simulink model "model"  (R2024b)
settings: Solver=ode4  StartTime=0.0  StopTime=1  FixedStep=0.0002  MaxStep=1e-4  RelTol=1e-3  EnableMultiTasking=on
undefined symbols (not defined in the file): rr, rs
libraries: spsRMSLib x1, simulink x1
settings Model: PacingRate=0.200000  Creator=jw  LastModifiedBy=tnt4
settings SolverCC: AlgebraicLoopSolver=TrustRegion
settings DataIOCC: LimitDataPoints=on  SaveFormat=Array  SignalLoggingSaveFormat=ModelDataLogs  ReturnWorkspaceOutputs=off
settings OptimizationCC: InitFltsAndDblsToZero=on  LifeSpan=inf
settings DebuggingCC: SaveWithParameterizedLinksMsg=none  UnderspecifiedInitializationDetection=Classic  MergeDetectMultiDrivingBlocksExec=none  SignalResolutionControl=TryResolveAllWithWarning  SolverPrmCheckMsg=warning  MultiTaskDSMMsg=warning  MultiTaskCondExecSysMsg=none  FcnCallInpInsideContextMsg=warning  UnconnectedInputMsg=warning  UnconnectedOutputMsg=warning  UnconnectedLineMsg=warning  SFUnexpectedBacktrackingDiag=warning  SFNoUnconditionalDefaultTransitionDiag=warning  SFExecutionAtInitializationDiag=none  ArithmeticOperatorsInVariantConditions=warning
settings HardwareCC: ProdBitPerPointer=32  ProdBitPerSizeT=32  ProdBitPerPtrDiffT=32  ProdLargestAtomicFloat=None  ProdIntDivRoundTo=Undefined  ProdEndianess=Unspecified  ProdWordSize=32  ProdHWDeviceType=32-bit Generic
settings ModelReferenceCC: EnableRefExpFcnMdlSchedulingChecks=on  PropagateSignalLabelsOutOfModel=off
settings SFSimCC: SimUseLocalCustomCode=off  CustomCodeUndefinedFunction=UseInterfaceOnly
settings RTWCC: RTWUseLocalCustomCode=off  GPUComputeCapability=3.5
settings CodeAppCC: StateflowObjectComments=on
settings GRTTargetCC: TargetFcnLib=ansi_tfl_tmw.mat  TargetLangStandard=C89/C90 (ANSI)  CombineOutputUpdateFcns=off  GRTInterface=on
settings ConfigComp: CovMetricSettings=dw  CovSaveCumulativeToWorkspaceVar=on  CovSaveSingleToWorkspaceVar=on  CovExternalEMLEnable=off

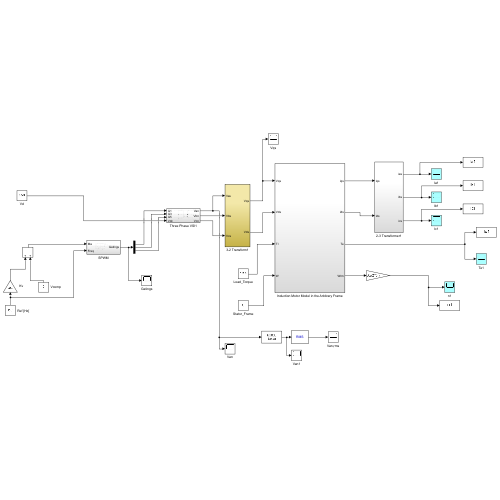
[thumbnail: Simulink's stored preview of the top-level diagram]
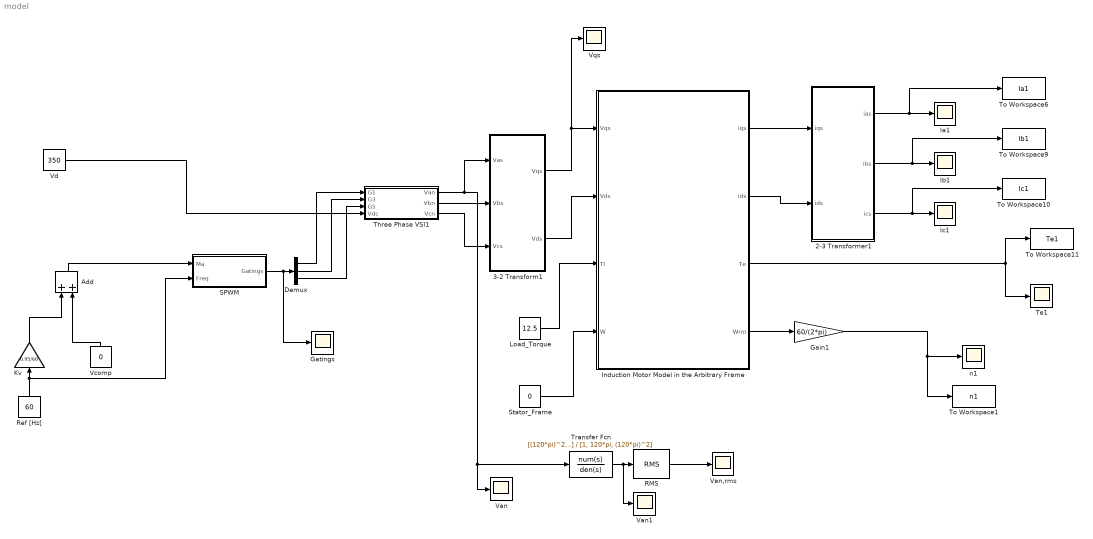
== system model ==
  2-3 Transformer1 : Subsystem
  3-2 Transform1 : Subsystem
  Add : Sum
  Demux : Demux  Outputs=3
  Gain1 : Gain  Gain=60/(2*pi)
  Gatings : Scope
  Ia1 : Scope
  Ib1 : Scope
  Ic1 : Scope
  Induction Motor Model in the Arbitrary Frame : Subsystem
  Kv : Gain  Gain=0.95/60
  Load_Torque : Constant  Value=12.5
  RMS : spsRMSLib/RMS  TrueRMS=on  Freq=60  RMSInit=0  Ts=0
  Ref [Hz[ : Constant  Value=60
  SPWM : Subsystem
  Stator_Frame : Constant  Value=0
  Te1 : Scope
  Three Phase VSI1 : Subsystem
  To Workspace1 : ToWorkspace  VariableName=n1  SampleTime=-1
  To Workspace10 : ToWorkspace  VariableName=Ic1  SampleTime=-1
  To Workspace11 : ToWorkspace  VariableName=Te1  SampleTime=-1
  To Workspace6 : ToWorkspace  VariableName=Ia1  SampleTime=-1
  To Workspace9 : ToWorkspace  VariableName=Ib1  SampleTime=-1
  Transfer Fcn : TransferFcn  Numerator=[(120*pi)^2]  Denominator=[1, 120*pi, (120*pi)^2]
  Van : Scope
  Van,rms : Scope
  Van1 : Scope
  Vcomp : Constant  Value=0
  Vd : Constant  Value=350
  Vqs : Scope
  n1 : Scope
  wires:
  Ref [Hz[/1 -> SPWM/2(Freq), Kv/1
  Kv/1 -> Add/1
  Vcomp/1 -> Add/2
  Add/1 -> SPWM/1(Ma)
  Vd/1 -> Three Phase VSI1/4(Vdc)
  SPWM/1(Gatings) -> Gatings/1, Demux/1
  Demux/1 -> Three Phase VSI1/1(G1)
  Demux/2 -> Three Phase VSI1/2(G3)
  Demux/3 -> Three Phase VSI1/3(G5)
  Three Phase VSI1/1(Van) -> Transfer Fcn/1, Van/1, 3-2 Transform1/1(Vas)
  Three Phase VSI1/2(Vbn) -> 3-2 Transform1/2(Vbs)
  Three Phase VSI1/3(Vcn) -> 3-2 Transform1/3(Vcs)
  3-2 Transform1/1(Vqs) -> Vqs/1, Induction Motor Model in the Arbitrary Frame/1(Vqs)
  3-2 Transform1/2(Vds) -> Induction Motor Model in the Arbitrary Frame/2(Vds)
  Stator_Frame/1 -> Induction Motor Model in the Arbitrary Frame/4(W)
  Load_Torque/1 -> Induction Motor Model in the Arbitrary Frame/3(Tl)
  Induction Motor Model in the Arbitrary Frame/1(iqs) -> 2-3 Transformer1/1(iqs)
  Induction Motor Model in the Arbitrary Frame/2(ids) -> 2-3 Transformer1/2(ids)
  Gain1/1 -> n1/1, To Workspace1/1
  Induction Motor Model in the Arbitrary Frame/4(Wrm) -> Gain1/1
  2-3 Transformer1/2(ibs) -> Ib1/1, To Workspace9/1
  2-3 Transformer1/3(ics) -> Ic1/1, To Workspace10/1
  2-3 Transformer1/1(ias) -> Ia1/1, To Workspace6/1
  Induction Motor Model in the Arbitrary Frame/3(Te) -> Te1/1, To Workspace11/1
  Transfer Fcn/1 -> Van1/1, RMS/1
  RMS/1 -> Van,rms/1

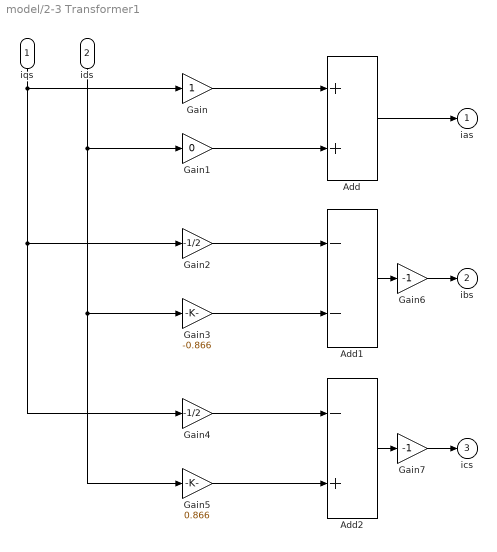
== system model/2-3 Transformer1 ==
  iqs : Inport
  ids : Inport  Port=2
  Add : Sum
  Add1 : Sum  Inputs=--
  Add2 : Sum  Inputs=-+
  Gain : Gain
  Gain1 : Gain  Gain=0
  Gain2 : Gain  Gain=-1/2
  Gain3 : Gain  Gain=-0.866
  Gain4 : Gain  Gain=-1/2
  Gain5 : Gain  Gain=0.866
  Gain6 : Gain  Gain=-1
  Gain7 : Gain  Gain=-1
  ias : Outport  InitialOutput=0  VectorParamsAs1DForOutWhenUnconnected=off
  ibs : Outport  Port=2  InitialOutput=0  VectorParamsAs1DForOutWhenUnconnected=off
  ics : Outport  Port=3  InitialOutput=0  VectorParamsAs1DForOutWhenUnconnected=off
  wires:
  Gain/1 -> Add/1
  Gain1/1 -> Add/2
  Gain2/1 -> Add1/1
  Gain3/1 -> Add1/2
  Gain4/1 -> Add2/1
  Gain5/1 -> Add2/2
  Add2/1 -> Gain7/1
  Add1/1 -> Gain6/1
  Add/1 -> ias/1
  iqs/1 -> Gain/1, Gain2/1, Gain4/1
  ids/1 -> Gain1/1, Gain3/1, Gain5/1
  Gain6/1 -> ibs/1
  Gain7/1 -> ics/1

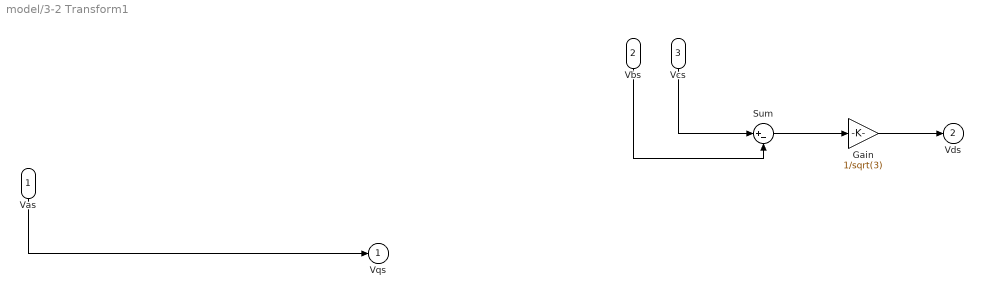
== system model/3-2 Transform1 ==
  Vas : Inport
  Vbs : Inport  Port=2
  Vcs : Inport  Port=3
  Gain : Gain  Gain=1/sqrt(3)
  Sum : Sum  Inputs=|+-
  Vqs : Outport  InitialOutput=0  VectorParamsAs1DForOutWhenUnconnected=off
  Vds : Outport  Port=2  InitialOutput=0  VectorParamsAs1DForOutWhenUnconnected=off
  wires:
  Vas/1 -> Vqs/1
  Vbs/1 -> Sum/2
  Vcs/1 -> Sum/1
  Sum/1 -> Gain/1
  Gain/1 -> Vds/1

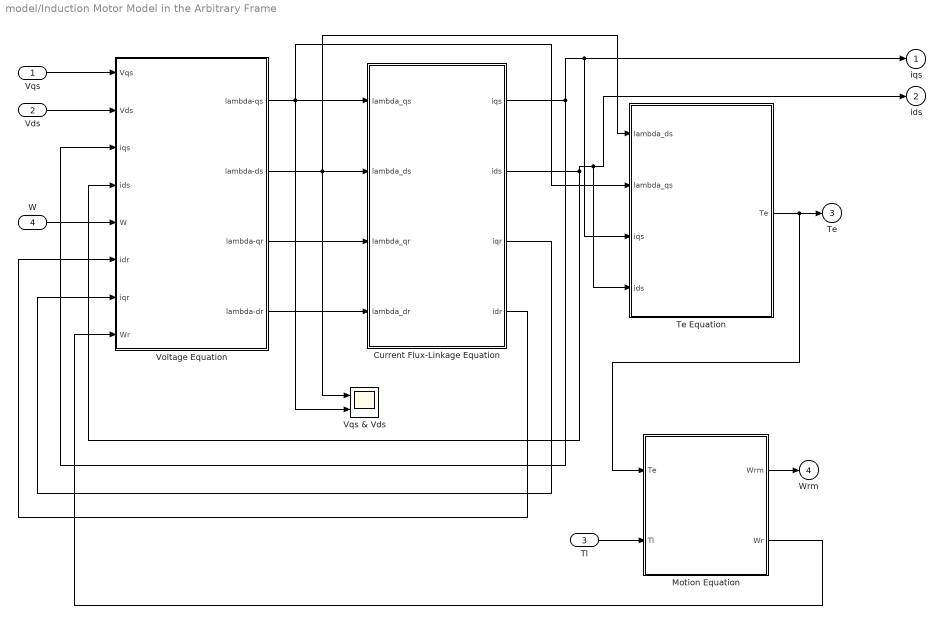
== system model/Induction Motor Model in the Arbitrary Frame ==
  Vqs : Inport
  Vds : Inport  Port=2
  Tl : Inport  Port=3
  W : Inport  Port=4
  Current Flux-Linkage Equation : Subsystem
  Motion Equation : Subsystem
  Te Equation : Subsystem
  Voltage Equation : Subsystem
  Vqs & Vds : Scope  NumInputPorts=2
  iqs : Outport  InitialOutput=0  VectorParamsAs1DForOutWhenUnconnected=off
  ids : Outport  Port=2  InitialOutput=0  VectorParamsAs1DForOutWhenUnconnected=off
  Te : Outport  Port=3  InitialOutput=0  VectorParamsAs1DForOutWhenUnconnected=off
  Wrm : Outport  Port=4  InitialOutput=0  VectorParamsAs1DForOutWhenUnconnected=off
  wires:
  Vqs/1 -> Voltage Equation/1(Vqs)
  Vds/1 -> Voltage Equation/2(Vds)
  Tl/1 -> Motion Equation/2(Tl)
  W/1 -> Voltage Equation/5(W)
  Te Equation/1(Te) -> Te/1, Motion Equation/1(Te)
  Current Flux-Linkage Equation/1(iqs) -> Voltage Equation/3(iqs), iqs/1, Te Equation/3(iqs)
  Current Flux-Linkage Equation/2(ids) -> Voltage Equation/4(ids), ids/1, Te Equation/4(ids)
  Current Flux-Linkage Equation/3(iqr) -> Voltage Equation/7(iqr)
  Voltage Equation/1(lambda-qs) -> Vqs & Vds/2, Current Flux-Linkage Equation/1(lambda_qs), Te Equation/2(lambda_qs)
  Voltage Equation/2(lambda-ds) -> Te Equation/1(lambda_ds), Vqs & Vds/1, Current Flux-Linkage Equation/2(lambda_ds)
  Voltage Equation/3(lambda-qr) -> Current Flux-Linkage Equation/3(lambda_qr)
  Voltage Equation/4(lambda-dr) -> Current Flux-Linkage Equation/4(lambda_dr)
  Current Flux-Linkage Equation/4(idr) -> Voltage Equation/6(idr)
  Motion Equation/2(Wr) -> Voltage Equation/8(Wr)
  Motion Equation/1(Wrm) -> Wrm/1

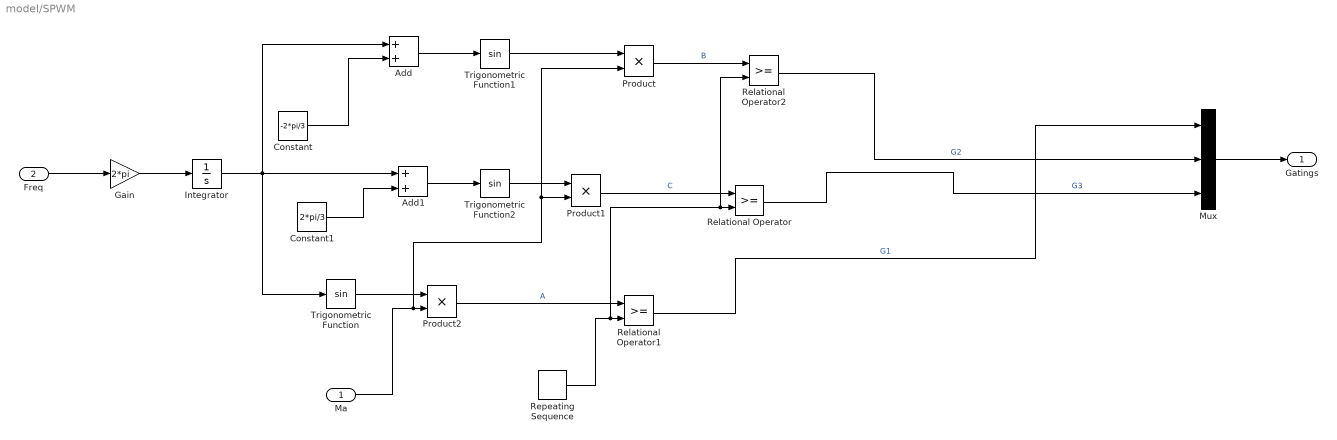
== system model/SPWM ==
  Ma : Inport
  Freq : Inport  Port=2
  Add : Sum
  Add1 : Sum
  Constant : Constant  Value=-2*pi/3
  Constant1 : Constant  Value=2*pi/3
  Gain : Gain  Gain=2*pi
  Integrator : Integrator
  Mux : Mux  Inputs=3
  Product : Product
  Product1 : Product
  Product2 : Product
  Relational Operator : RelationalOperator  OutDataTypeStr=boolean  RndMeth=Simplest  InputSameDT=off
  Relational Operator1 : RelationalOperator  OutDataTypeStr=boolean  RndMeth=Simplest  InputSameDT=off
  Relational Operator2 : RelationalOperator  OutDataTypeStr=boolean  RndMeth=Simplest  InputSameDT=off
  Repeating Sequence : simulink/Sources/Repeating Sequence  rep_seq_t=[0, 0.5/2000, 1/2000]  rep_seq_y=[-1, 1, -1]
  Trigonometric Function : Trigonometry
  Trigonometric Function1 : Trigonometry
  Trigonometric Function2 : Trigonometry
  Gatings : Outport
  wires:
  Integrator/1 -> Add1/1, Add/1, Trigonometric Function/1
  Ma/1 -> Product1/2, Product/2, Product2/2
  Gain/1 -> Integrator/1
  Add/1 -> Trigonometric Function1/1
  Trigonometric Function1/1 -> Product/1
  Trigonometric Function/1 -> Product2/1
  Add1/1 -> Trigonometric Function2/1
  Trigonometric Function2/1 -> Product1/1
  Constant/1 -> Add/2
  Constant1/1 -> Add1/2
  Freq/1 -> Gain/1
  Product/1 -> Relational Operator2/1  "B"
  Product1/1 -> Relational Operator/1  "C"
  Product2/1 -> Relational Operator1/1  "A"
  Repeating Sequence/1 -> Relational Operator2/2, Relational Operator/2, Relational Operator1/2
  Relational Operator1/1 -> Mux/1  "G1"
  Relational Operator2/1 -> Mux/2  "G2"
  Relational Operator/1 -> Mux/3  "G3"
  Mux/1 -> Gatings/1

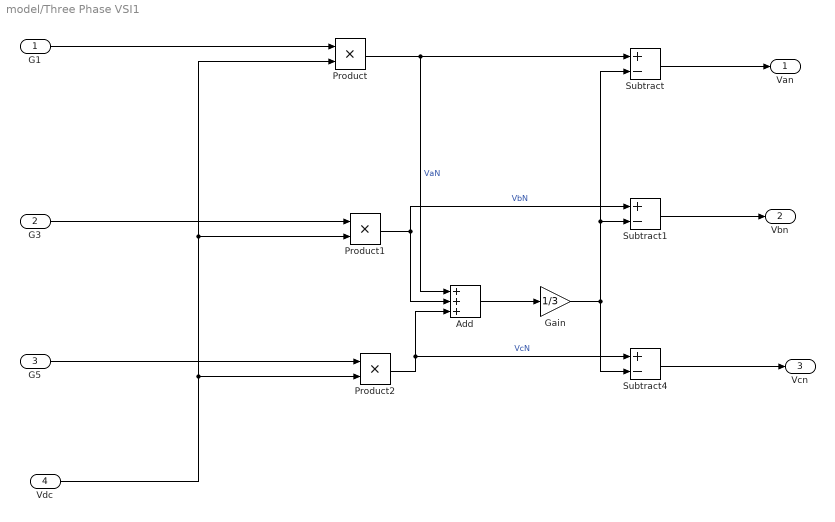
== system model/Three Phase VSI1 ==
  G1 : Inport
  G3 : Inport  Port=2
  G5 : Inport  Port=3
  Vdc : Inport  Port=4
  Add : Sum  Inputs=+++
  Gain : Gain  Gain=1/3
  Product : Product
  Product1 : Product
  Product2 : Product
  Subtract : Sum  Inputs=+-
  Subtract1 : Sum  Inputs=+-
  Subtract4 : Sum  Inputs=+-
  Van : Outport
  Vbn : Outport  Port=2
  Vcn : Outport  Port=3
  wires:
  G1/1 -> Product/1
  G3/1 -> Product1/1
  G5/1 -> Product2/1
  Vdc/1 -> Product2/2, Product1/2, Product/2
  Product/1 -> Subtract/1, Add/1  "VaN"
  Product1/1 -> Add/2, Subtract1/1  "VbN"
  Product2/1 -> Add/3, Subtract4/1  "VcN"
  Add/1 -> Gain/1
  Gain/1 -> Subtract4/2, Subtract1/2, Subtract/2
  Subtract/1 -> Van/1
  Subtract1/1 -> Vbn/1
  Subtract4/1 -> Vcn/1

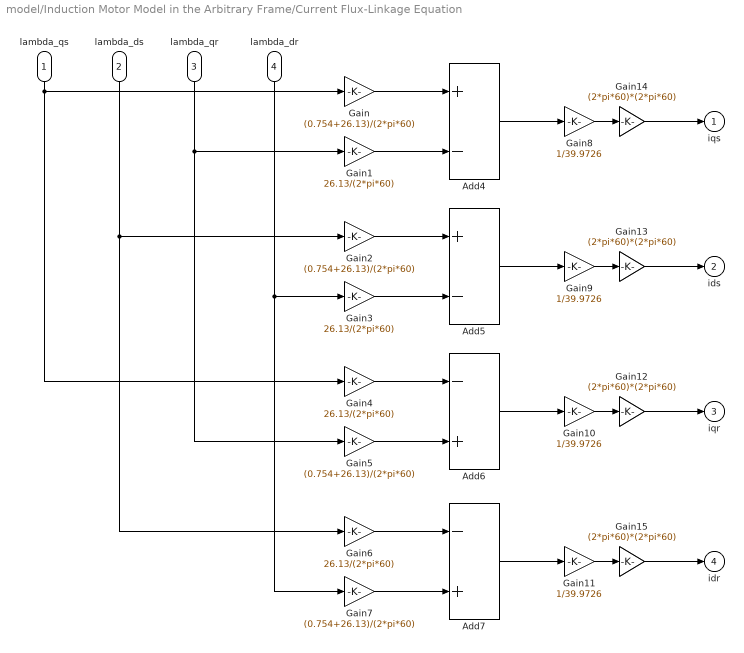
== system model/Induction Motor Model in the Arbitrary Frame/Current Flux-Linkage Equation ==
  lambda_qs : Inport
  lambda_ds : Inport  Port=2
  lambda_qr : Inport  Port=3
  lambda_dr : Inport  Port=4
  Add4 : Sum  Inputs=+-
  Add5 : Sum  Inputs=+-
  Add6 : Sum  Inputs=-+
  Add7 : Sum  Inputs=-+
  Gain{,2,5,7} (4 alike) : Gain  Gain=(0.754+26.13)/(2*pi*60)
  Gain{1,3..4,6} (4 alike) : Gain  Gain=26.13/(2*pi*60)
  Gain{8..11} (4 alike) : Gain  Gain=1/39.9726
  Gain{12..15} (4 alike) : Gain  Gain=(2*pi*60)*(2*pi*60)
  iqs : Outport  InitialOutput=0  VectorParamsAs1DForOutWhenUnconnected=off
  ids : Outport  Port=2  InitialOutput=0  VectorParamsAs1DForOutWhenUnconnected=off
  iqr : Outport  Port=3  InitialOutput=0  VectorParamsAs1DForOutWhenUnconnected=off
  idr : Outport  Port=4  InitialOutput=0  VectorParamsAs1DForOutWhenUnconnected=off
  wires:
  Gain1/1 -> Add4/2
  Gain/1 -> Add4/1
  Gain2/1 -> Add5/1
  Gain3/1 -> Add5/2
  Gain4/1 -> Add6/1
  Gain5/1 -> Add6/2
  Gain6/1 -> Add7/1
  Gain7/1 -> Add7/2
  Add4/1 -> Gain8/1
  Add5/1 -> Gain9/1
  Add6/1 -> Gain10/1
  Add7/1 -> Gain11/1
  lambda_qs/1 -> Gain/1, Gain4/1
  lambda_qr/1 -> Gain1/1, Gain5/1
  Gain10/1 -> Gain12/1
  Gain9/1 -> Gain13/1
  Gain8/1 -> Gain14/1
  Gain11/1 -> Gain15/1
  lambda_ds/1 -> Gain2/1, Gain6/1
  lambda_dr/1 -> Gain3/1, Gain7/1
  Gain14/1 -> iqs/1
  Gain13/1 -> ids/1
  Gain12/1 -> iqr/1
  Gain15/1 -> idr/1

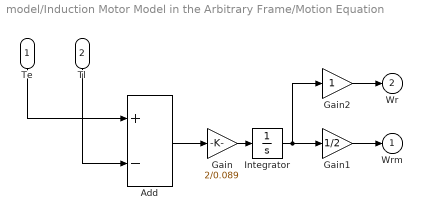
== system model/Induction Motor Model in the Arbitrary Frame/Motion Equation ==
  Te : Inport
  Tl : Inport  Port=2
  Add : Sum  Inputs=+-
  Gain : Gain  Gain=2/0.089
  Gain1 : Gain  Gain=1/2
  Gain2 : Gain
  Integrator : Integrator
  Wrm : Outport  InitialOutput=0  VectorParamsAs1DForOutWhenUnconnected=off
  Wr : Outport  Port=2  InitialOutput=0  VectorParamsAs1DForOutWhenUnconnected=off
  wires:
  Te/1 -> Add/1
  Tl/1 -> Add/2
  Gain/1 -> Integrator/1
  Add/1 -> Gain/1
  Integrator/1 -> Gain2/1, Gain1/1
  Gain2/1 -> Wr/1
  Gain1/1 -> Wrm/1

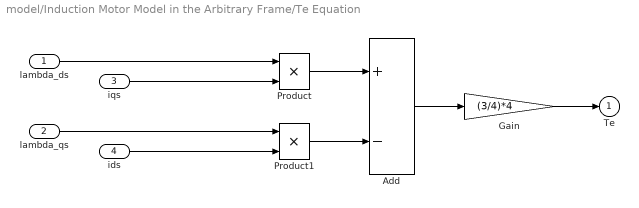
== system model/Induction Motor Model in the Arbitrary Frame/Te Equation ==
  lambda_ds : Inport
  lambda_qs : Inport  Port=2
  iqs : Inport  Port=3
  ids : Inport  Port=4
  Add : Sum  Inputs=+-
  Gain : Gain  Gain=(3/4)*4
  Product : Product  RndMeth=Zero
  Product1 : Product  RndMeth=Zero
  Te : Outport  InitialOutput=0  VectorParamsAs1DForOutWhenUnconnected=off
  wires:
  Gain/1 -> Te/1
  Add/1 -> Gain/1
  lambda_ds/1 -> Product/1
  iqs/1 -> Product/2
  lambda_qs/1 -> Product1/1
  ids/1 -> Product1/2
  Product/1 -> Add/1
  Product1/1 -> Add/2

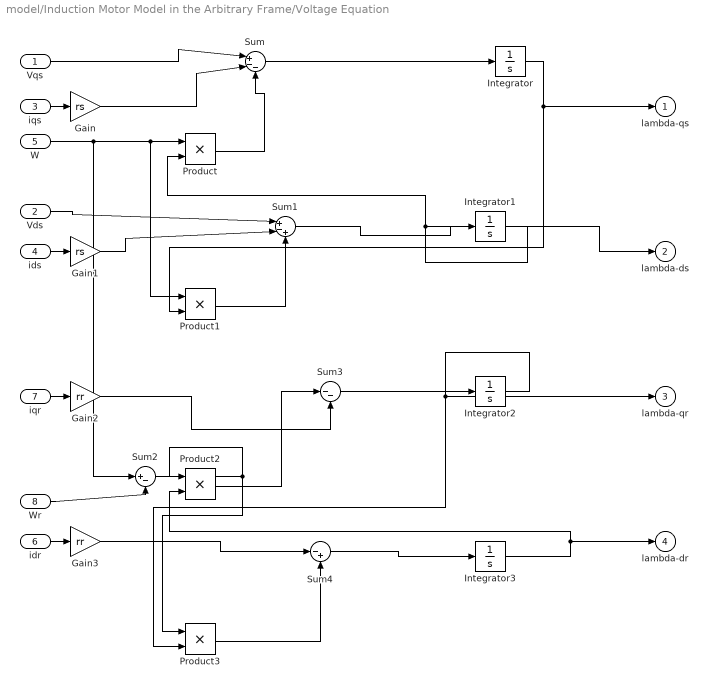
== system model/Induction Motor Model in the Arbitrary Frame/Voltage Equation ==
  Vqs : Inport
  Vds : Inport  Port=2
  iqs : Inport  Port=3
  ids : Inport  Port=4
  W : Inport  Port=5
  idr : Inport  Port=6
  iqr : Inport  Port=7
  Wr : Inport  Port=8
  Gain : Gain  Gain=rs
  Gain1 : Gain  Gain=rs
  Gain2 : Gain  Gain=rr
  Gain3 : Gain  Gain=rr
  Integrator{,1..3} (4 alike) : Integrator
  Product{,1..3} (4 alike) : Product
  Sum : Sum  Inputs=|+--
  Sum1 : Sum  Inputs=|+-+
  Sum2 : Sum  Inputs=|+-
  Sum3 : Sum  Inputs=|--
  Sum4 : Sum  Inputs=|-+
  lambda-qs : Outport  InitialOutput=0  VectorParamsAs1DForOutWhenUnconnected=off
  lambda-ds : Outport  Port=2  InitialOutput=0  VectorParamsAs1DForOutWhenUnconnected=off
  lambda-qr : Outport  Port=3  InitialOutput=0  VectorParamsAs1DForOutWhenUnconnected=off
  lambda-dr : Outport  Port=4  InitialOutput=0  VectorParamsAs1DForOutWhenUnconnected=off
  wires:
  iqs/1 -> Gain/1
  Vqs/1 -> Sum/1
  Gain/1 -> Sum/2
  W/1 -> Sum2/1, Product1/1, Product/1
  Product/1 -> Sum/3
  Sum/1 -> Integrator/1
  Integrator/1 -> Product1/2, lambda-qs/1
  Vds/1 -> Sum1/1
  ids/1 -> Gain1/1
  Gain1/1 -> Sum1/2
  Product1/1 -> Sum1/3
  Sum1/1 -> Integrator1/1
  Integrator1/1 -> Product/2, lambda-ds/1
  Wr/1 -> Sum2/2
  iqr/1 -> Gain2/1
  Gain2/1 -> Sum3/2
  Sum2/1 -> Product3/1, Product2/1
  Product2/1 -> Sum3/1
  Sum3/1 -> Integrator2/1
  Integrator2/1 -> Product3/2, lambda-qr/1
  idr/1 -> Gain3/1
  Gain3/1 -> Sum4/1
  Product3/1 -> Sum4/2
  Integrator3/1 -> Product2/2, lambda-dr/1
  Sum4/1 -> Integrator3/1
